simulink model "euler_ZXY_model"  (R2023b)
settings: Solver=FixedStepAuto  StartTime=0.0  StopTime=fs  FixedStep=ts  MaxStep=1e-4  RelTol=1e-3
undefined symbols (not defined in the file): alpha, alpha_1, alpha_2, alpha_d, e1, e2, e3, eta_0, eta_dot_0, f_max, g, gamma, gamma_d, gamma_e, gamma_u, gamma_x, gamma_x1, gamma_x2, J, k_3, k_beta, k_d_gamma, K_p, k_p_gamma, k_R, m, p_0, p_d_0, p_dot_0, p_dot_zmax, r, ts, y_c, z_c, z_dot_max, z_max
libraries: eeGeneralControl x8, slctrl_constraint x6, simulink x2, rbm3d x1, simulink_extras x1
(part 2 of 2)

== system euler_ZXY_model/dynamics/回転方向の運動方程式/Subsystem ==
  M : Inport
  Psi : Inport  Port=2
  tau^b : Inport  Port=3
  C : Inport  Port=4
  eta_dot : Inport  Port=5
  Constant : Constant  Value=e1
  Matrix Multiply : Product  Inputs=3  Multiplication=Matrix(*)
  Matrix Multiply1 : Product  Inputs=3  Multiplication=Matrix(*)
  Matrix Multiply2 : Product  Multiplication=Matrix(*)
  Matrix Multiply3 : Product  Multiplication=Matrix(*)
  Matrix Multiply4 : Product  Multiplication=Matrix(*)
  Product : Product  Inputs=/  Multiplication=Matrix(*)
  Product1 : Product  Inputs=/  Multiplication=Matrix(*)
  Sum : Sum  Inputs=|+-
  Transpose : Math  Operator=transpose
  Transpose1 : Math  Operator=transpose
  lambda_3 : Outport
  wires:
  Constant/1 -> Matrix Multiply/3, Transpose/1
  Transpose/1 -> Matrix Multiply/1, Matrix Multiply1/2
  M/1 -> Product/1
  Product/1 -> Matrix Multiply1/3, Matrix Multiply/2
  Matrix Multiply/1 -> Product1/1
  Product1/1 -> Matrix Multiply1/1
  Matrix Multiply1/1 -> Matrix Multiply2/1
  Matrix Multiply2/1 -> lambda_3/1
  Psi/1 -> Transpose1/1
  Transpose1/1 -> Matrix Multiply3/1
  tau^b/1 -> Matrix Multiply3/2
  Matrix Multiply3/1 -> Sum/1
  C/1 -> Matrix Multiply4/1
  eta_dot/1 -> Matrix Multiply4/2
  Matrix Multiply4/1 -> Sum/2
  Sum/1 -> Matrix Multiply2/2

== system euler_ZXY_model/dynamics/回転方向の運動方程式/eta to R_SO(2) ==
  eta : Inport
  Cos1 : Trigonometry  Operator=cos
  Cos2 : Trigonometry  Operator=cos
  Gain : Gain  Gain=-1
  Matrix Concatenate : Concatenate  Mode=Multidimensional array  ConcatenateDimension=2
  Mux1 : Mux  Inputs=2
  Mux2 : Mux  Inputs=2
  Selector : Selector  InputPortWidth=3  IndexOptions=Index vector (dialog)  Indices=[2]  OutputSizes=1
  Sin1 : Trigonometry
  Sin2 : Trigonometry
  attitude_state : Outport
  wires:
  eta/1 -> Selector/1
  Cos2/1 -> Mux2/2
  Matrix Concatenate/1 -> attitude_state/1
  Mux2/1 -> Matrix Concatenate/2
  Mux1/1 -> Matrix Concatenate/1
  Gain/1 -> Sin2/1
  Cos1/1 -> Mux1/1
  Sin2/1 -> Mux2/1
  Sin1/1 -> Mux1/2
  Selector/1 -> Cos2/1, Gain/1, Cos1/1, Sin1/1  "beta"

== system euler_ZXY_model/Attitude Controller/beta_controller/r_beta/R_tilde ==
  R_d : Inport
  R : Inport  Port=2
  Matrix Multiply : Product  Multiplication=Matrix(*)
  Transpose : Math  Operator=transpose
  R_tilde : Outport
  wires:
  R_d/1 -> Transpose/1
  Transpose/1 -> Matrix Multiply/1
  R/1 -> Matrix Multiply/2
  Matrix Multiply/1 -> R_tilde/1

== system euler_ZXY_model/Attitude Controller/beta_controller/r_beta/r_beta_d ==
  R_d : Inport
  R_d_dot : Inport  Port=2
  Matrix Multiply : Product  Multiplication=Matrix(*)
  Selector : Selector  NumberOfDimensions=2  InputPortWidth=3  IndexOptions=Index vector (dialog),Index vector (dialog)  Indices=[2],1  OutputSizes=1,1
  Transpose : Math  Operator=transpose
  "r_{beta_d}" : Outport
  wires:
  R_d/1 -> Transpose/1
  Transpose/1 -> Matrix Multiply/1
  R_d_dot/1 -> Matrix Multiply/2
  Matrix Multiply/1 -> Selector/1
  Selector/1 -> "r_{beta_d}"/1

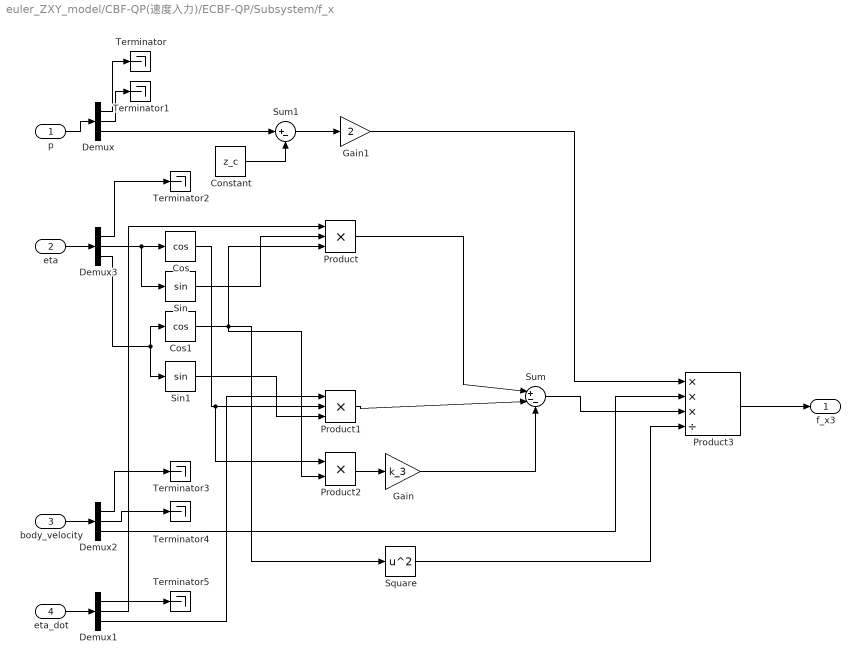
== system euler_ZXY_model/CBF-QP(速度入力)/ECBF-QP/Subsystem/f_x ==
  p : Inport
  eta : Inport  Port=2
  body_velocity : Inport  Port=3
  eta_dot : Inport  Port=4
  Constant : Constant  Value=z_c
  Cos : Trigonometry  Operator=cos
  Cos1 : Trigonometry  Operator=cos
  Demux{,1..3} (4 alike) : Demux  Outputs=3
  Gain : Gain  Gain=k_3
  Gain1 : Gain  Gain=2
  Product : Product  Inputs=3
  Product1 : Product  Inputs=3
  Product2 : Product
  Product3 : Product  Inputs=***/
  Sin : Trigonometry
  Sin1 : Trigonometry
  Square : Math  Operator=square
  Sum : Sum  Inputs=|+--
  Sum1 : Sum  Inputs=|+-
  Terminator{,1..5} (6 alike) : Terminator
  f_x3 : Outport
  wires:
  p/1 -> Demux/1
  Demux/1 -> Terminator/1
  Demux/2 -> Terminator1/1
  eta_dot/1 -> Demux1/1
  body_velocity/1 -> Demux2/1
  eta/1 -> Demux3/1
  Demux3/2 -> Sin/1, Cos/1
  Demux3/3 -> Sin1/1, Cos1/1
  Sin/1 -> Product/2
  Cos1/1 -> Square/1, Product/3, Product2/2
  Demux3/1 -> Terminator2/1
  Demux1/2 -> Product/1
  Demux1/3 -> Product1/1
  Sin1/1 -> Product1/3
  Cos/1 -> Product2/1, Product1/2
  Product2/1 -> Gain/1
  Product1/1 -> Sum/2
  Gain/1 -> Sum/3
  Product/1 -> Sum/1
  Demux/3 -> Sum1/1
  Constant/1 -> Sum1/2
  Sum1/1 -> Gain1/1
  Gain1/1 -> Product3/1
  Demux2/3 -> Product3/2
  Sum/1 -> Product3/3
  Square/1 -> Product3/4
  Product3/1 -> f_x3/1
  Demux2/1 -> Terminator3/1
  Demux2/2 -> Terminator4/1
  Demux1/1 -> Terminator5/1

== system euler_ZXY_model/CBF-QP(速度入力)/ECBF-QP/Subsystem/f_x1 ==
  p_dot : Inport
  Demux : Demux  Outputs=3
  Gain : Gain  Gain=-2
  Square : Math  Operator=square
  Square1 : Math  Operator=square
  Sum : Sum  Inputs=|++
  Terminator : Terminator
  f_x1 : Outport
  wires:
  p_dot/1 -> Demux/1
  Demux/1 -> Terminator/1
  Demux/2 -> Square/1
  Demux/3 -> Square1/1
  Square/1 -> Sum/1
  Square1/1 -> Sum/2
  Sum/1 -> Gain/1
  Gain/1 -> f_x1/1

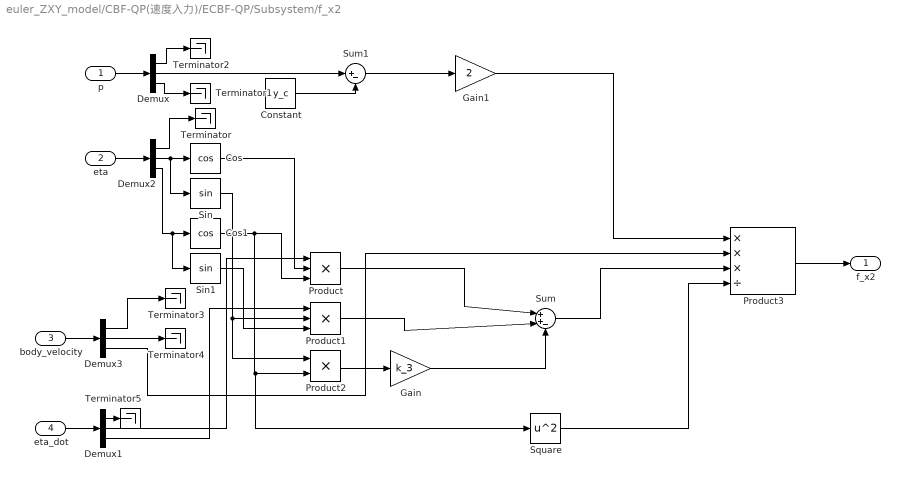
== system euler_ZXY_model/CBF-QP(速度入力)/ECBF-QP/Subsystem/f_x2 ==
  p : Inport
  eta : Inport  Port=2
  body_velocity : Inport  Port=3
  eta_dot : Inport  Port=4
  Constant : Constant  Value=y_c
  Cos : Trigonometry  Operator=cos
  Cos1 : Trigonometry  Operator=cos
  Demux{,1..3} (4 alike) : Demux  Outputs=3
  Gain : Gain  Gain=k_3
  Gain1 : Gain  Gain=2
  Product : Product  Inputs=3
  Product1 : Product  Inputs=3
  Product2 : Product
  Product3 : Product  Inputs=***/
  Sin : Trigonometry
  Sin1 : Trigonometry
  Square : Math  Operator=square
  Sum : Sum  Inputs=|++-
  Sum1 : Sum  Inputs=|+-
  Terminator{,1..5} (6 alike) : Terminator
  f_x2 : Outport
  wires:
  p/1 -> Demux/1
  eta_dot/1 -> Demux1/1
  eta/1 -> Demux2/1
  body_velocity/1 -> Demux3/1
  Demux2/2 -> Sin/1, Cos/1
  Demux2/3 -> Sin1/1, Cos1/1
  Demux2/1 -> Terminator/1
  Cos1/1 -> Square/1, Product2/2, Product/3
  Cos/1 -> Product/2
  Sin1/1 -> Product1/3
  Sin/1 -> Product2/1, Product1/2
  Product2/1 -> Gain/1
  Gain/1 -> Sum/3
  Product1/1 -> Sum/2
  Product/1 -> Sum/1
  Demux/3 -> Terminator1/1
  Demux/1 -> Terminator2/1
  Demux/2 -> Sum1/1
  Constant/1 -> Sum1/2
  Sum1/1 -> Gain1/1
  Gain1/1 -> Product3/1
  Demux1/2 -> Product/1
  Demux1/3 -> Product1/1
  Demux3/3 -> Product3/2
  Sum/1 -> Product3/3
  Square/1 -> Product3/4
  Product3/1 -> f_x2/1
  Demux3/1 -> Terminator3/1
  Demux3/2 -> Terminator4/1
  Demux1/1 -> Terminator5/1

== system euler_ZXY_model/CBF-QP(速度入力)/ECBF-QP/c/Subsystem ==
  p : Inport
  p_dot : Inport  Port=2
  Constant : Constant  Value=y_c
  Constant1 : Constant  Value=z_c
  Demux : Demux  Outputs=3
  Demux1 : Demux  Outputs=3
  Gain : Gain  Gain=2
  Product : Product
  Product1 : Product
  Sum : Sum  Inputs=|+-
  Sum1 : Sum  Inputs=|+-
  Sum2 : Sum  Inputs=|++
  Terminator : Terminator
  Terminator1 : Terminator
  h_dot : Outport
  wires:
  p/1 -> Demux/1
  p_dot/1 -> Demux1/1
  Demux/1 -> Terminator/1
  Demux1/1 -> Terminator1/1
  Demux/2 -> Sum/1
  Constant/1 -> Sum/2
  Sum/1 -> Product/1
  Demux1/2 -> Product/2
  Gain/1 -> h_dot/1
  Product/1 -> Sum2/1
  Sum2/1 -> Gain/1
  Demux/3 -> Sum1/1
  Sum1/1 -> Product1/1
  Constant1/1 -> Sum1/2
  Demux1/3 -> Product1/2
  Product1/1 -> Sum2/2

== system euler_ZXY_model/CBF-QP(速度入力)/ECBF-QP/c/h ==
  p : Inport
  Constant : Constant  Value=y_c
  Constant1 : Constant  Value=r
  Constant2 : Constant  Value=z_c
  Demux : Demux  Outputs=3
  Square : Math  Operator=square
  Square1 : Math  Operator=square
  Sum : Sum  Inputs=|+-
  Sum1 : Sum  Inputs=|+-
  Sum2 : Sum  Inputs=|++-
  Terminator : Terminator
  h : Outport
  wires:
  p/1 -> Demux/1
  Demux/2 -> Sum/1
  Demux/3 -> Sum1/1
  Constant1/1 -> Sum2/3
  Sum2/1 -> h/1
  Sum/1 -> Square/1
  Sum1/1 -> Square1/1
  Square/1 -> Sum2/1
  Square1/1 -> Sum2/2
  Constant/1 -> Sum/2
  Constant2/1 -> Sum1/2
  Demux/1 -> Terminator/1

== system euler_ZXY_model/CBF-QP(速度入力)/ECBF-QP_rengo_ver./c/h ==
  p : Inport
  Constant : Constant  Value=y_c
  Constant1 : Constant  Value=r
  Constant2 : Constant  Value=z_c
  Demux : Demux  Outputs=3
  Square : Math  Operator=square
  Square1 : Math  Operator=square
  Sum : Sum  Inputs=|+-
  Sum1 : Sum  Inputs=|+-
  Sum2 : Sum  Inputs=|++-
  Terminator : Terminator
  h : Outport
  wires:
  p/1 -> Demux/1
  Demux/2 -> Sum/1
  Demux/3 -> Sum1/1
  Constant1/1 -> Sum2/3
  Sum2/1 -> h/1
  Sum/1 -> Square/1
  Sum1/1 -> Square1/1
  Square/1 -> Sum2/1
  Square1/1 -> Sum2/2
  Constant/1 -> Sum/2
  Constant2/1 -> Sum1/2
  Demux/1 -> Terminator/1

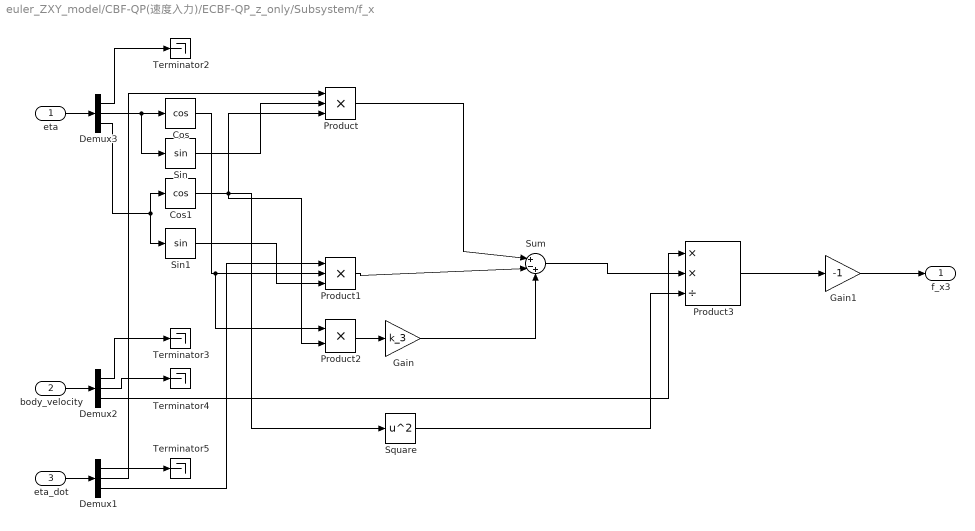
== system euler_ZXY_model/CBF-QP(速度入力)/ECBF-QP_z_only/Subsystem/f_x ==
  eta : Inport
  body_velocity : Inport  Port=2
  eta_dot : Inport  Port=3
  Cos : Trigonometry  Operator=cos
  Cos1 : Trigonometry  Operator=cos
  Demux1 : Demux  Outputs=3
  Demux2 : Demux  Outputs=3
  Demux3 : Demux  Outputs=3
  Gain : Gain  Gain=k_3
  Gain1 : Gain  Gain=-1
  Product : Product  Inputs=3
  Product1 : Product  Inputs=3
  Product2 : Product
  Product3 : Product  Inputs=**/
  Sin : Trigonometry
  Sin1 : Trigonometry
  Square : Math  Operator=square
  Sum : Sum  Inputs=|+-+
  Terminator{2..5} (4 alike) : Terminator
  f_x3 : Outport
  wires:
  eta_dot/1 -> Demux1/1
  body_velocity/1 -> Demux2/1
  eta/1 -> Demux3/1
  Demux3/2 -> Sin/1, Cos/1
  Demux3/3 -> Sin1/1, Cos1/1
  Sin/1 -> Product/2
  Cos1/1 -> Square/1, Product/3, Product2/2
  Demux3/1 -> Terminator2/1
  Demux1/2 -> Product/1
  Demux1/3 -> Product1/1
  Sin1/1 -> Product1/3
  Cos/1 -> Product2/1, Product1/2
  Product2/1 -> Gain/1
  Product1/1 -> Sum/2
  Gain/1 -> Sum/3
  Product/1 -> Sum/1
  Demux2/3 -> Product3/1
  Sum/1 -> Product3/2
  Square/1 -> Product3/3
  Demux2/1 -> Terminator3/1
  Demux2/2 -> Terminator4/1
  Demux1/1 -> Terminator5/1
  Product3/1 -> Gain1/1
  Gain1/1 -> f_x3/1

== system euler_ZXY_model/CBF-QP(速度入力)/ECBF-QP_z_only/c/Subsystem ==
  p_dot : Inport
  Demux1 : Demux  Outputs=3
  Gain : Gain  Gain=-1
  Terminator1 : Terminator
  Terminator2 : Terminator
  h_dot : Outport
  wires:
  p_dot/1 -> Demux1/1
  Demux1/1 -> Terminator1/1
  Gain/1 -> h_dot/1
  Demux1/2 -> Terminator2/1
  Demux1/3 -> Gain/1

== system euler_ZXY_model/CBF-QP(速度入力)/ECBF-QP_z_only/c/h ==
  p : Inport
  Constant2 : Constant  Value=z_c
  Demux : Demux  Outputs=3
  Gain : Gain  Gain=-1
  Sum1 : Sum  Inputs=|+-
  Terminator : Terminator
  Terminator1 : Terminator
  h : Outport
  wires:
  p/1 -> Demux/1
  Demux/2 -> Terminator1/1
  Demux/3 -> Sum1/1
  Gain/1 -> h/1
  Sum1/1 -> Gain/1
  Constant2/1 -> Sum1/2
  Demux/1 -> Terminator/1

== system euler_ZXY_model/dynamics/並進方向の運動方程式/B/Subsystem ==
  R : Inport
  Constant1 : Constant  Value=0
  Selector : Selector  NumberOfDimensions=2  InputPortWidth=3  IndexOptions=Index vector (dialog),Index vector (dialog)  Indices=[2],[2]  OutputSizes=1,1
  Selector1 : Selector  NumberOfDimensions=2  InputPortWidth=3  IndexOptions=Index vector (dialog),Index vector (dialog)  Indices=[3],[2]  OutputSizes=1,1
  Transpose : Math  Operator=transpose
  Vector Concatenate : Concatenate  NumInputs=3
  A : Outport
  wires:
  R/1 -> Selector1/1, Selector/1
  Selector/1 -> Vector Concatenate/2
  Selector1/1 -> Vector Concatenate/3
  Constant1/1 -> Vector Concatenate/1
  Vector Concatenate/1 -> Transpose/1
  Transpose/1 -> A/1

== system euler_ZXY_model/dynamics/並進方向の運動方程式/Rotation matrix_ZXY/R1 ==
  In1 : Inport
  Cos : Trigonometry  Operator=cos
  Cos1 : Trigonometry  Operator=cos
  Cos2 : Trigonometry  Operator=cos
  Demux : Demux  Outputs=3
  Gain : Gain  Gain=-1
  Matrix Concatenate : Concatenate  NumInputs=3
  Product : Product
  Product1 : Product  Inputs=3
  Product2 : Product
  Product3 : Product  Inputs=3
  Product4 : Product
  Sin : Trigonometry
  Sin1 : Trigonometry
  Sin2 : Trigonometry
  Sum : Sum  Inputs=|+-
  Sum1 : Sum  Inputs=|++
  Out1 : Outport  VectorParamsAs1DForOutWhenUnconnected=off
  wires:
  Matrix Concatenate/1 -> Out1/1
  In1/1 -> Demux/1
  Demux/3 -> Sin/1, Cos/1
  Demux/2 -> Sin1/1, Cos1/1
  Demux/1 -> Cos2/1, Sin2/1
  Cos2/1 -> Product3/1, Product/1
  Cos/1 -> Product2/2, Product/2
  Product/1 -> Sum/1
  Sin2/1 -> Product2/1, Product1/1
  Sin1/1 -> Product3/2, Product1/2
  Sin/1 -> Product3/3, Product1/3, Product4/2
  Product1/1 -> Sum/2
  Product2/1 -> Sum1/1
  Product3/1 -> Sum1/2
  Cos1/1 -> Product4/1
  Product4/1 -> Gain/1
  Sum1/1 -> Matrix Concatenate/2
  Gain/1 -> Matrix Concatenate/3
  Sum/1 -> Matrix Concatenate/1

== system euler_ZXY_model/dynamics/並進方向の運動方程式/Rotation matrix_ZXY/R2 ==
  In1 : Inport
  Cos1 : Trigonometry  Operator=cos
  Cos2 : Trigonometry  Operator=cos
  Demux : Demux  Outputs=3
  Gain : Gain  Gain=-1
  Matrix Concatenate : Concatenate  NumInputs=3
  Product : Product
  Product1 : Product
  Sin1 : Trigonometry
  Sin2 : Trigonometry
  Terminator : Terminator
  Out1 : Outport  VectorParamsAs1DForOutWhenUnconnected=off
  wires:
  In1/1 -> Demux/1
  Demux/2 -> Cos1/1, Sin1/1
  Matrix Concatenate/1 -> Out1/1
  Demux/1 -> Cos2/1, Sin2/1
  Sin2/1 -> Product/1
  Cos1/1 -> Product/2, Product1/2
  Product/1 -> Gain/1
  Cos2/1 -> Product1/1
  Gain/1 -> Matrix Concatenate/1
  Product1/1 -> Matrix Concatenate/2
  Sin1/1 -> Matrix Concatenate/3
  Demux/3 -> Terminator/1

== system euler_ZXY_model/dynamics/並進方向の運動方程式/Rotation matrix_ZXY/R3 ==
  In1 : Inport
  Cos1 : Trigonometry  Operator=cos
  Cos2 : Trigonometry  Operator=cos
  Cos3 : Trigonometry  Operator=cos
  Demux : Demux  Outputs=3
  Matrix Concatenate : Concatenate  NumInputs=3
  Product : Product
  Product1 : Product  Inputs=3
  Product2 : Product
  Product3 : Product  Inputs=3
  Product4 : Product
  Sin1 : Trigonometry
  Sin2 : Trigonometry
  Sin3 : Trigonometry
  Sum : Sum  Inputs=|++
  Sum1 : Sum  Inputs=|+-
  Out1 : Outport  VectorParamsAs1DForOutWhenUnconnected=off
  wires:
  Matrix Concatenate/1 -> Out1/1
  Demux/2 -> Sin1/1, Cos1/1
  Demux/3 -> Sin2/1, Cos2/1
  In1/1 -> Demux/1
  Cos2/1 -> Product4/2, Product3/3, Product1/3
  Demux/1 -> Cos3/1, Sin3/1
  Cos3/1 -> Product3/1, Product/1
  Sin2/1 -> Product2/2, Product/2
  Product/1 -> Sum/1
  Sin3/1 -> Product2/1, Product1/1
  Sin1/1 -> Product3/2, Product1/2
  Product1/1 -> Sum/2
  Product2/1 -> Sum1/1
  Product3/1 -> Sum1/2
  Cos1/1 -> Product4/1
  Sum/1 -> Matrix Concatenate/1
  Sum1/1 -> Matrix Concatenate/2
  Product4/1 -> Matrix Concatenate/3

== system euler_ZXY_model/dynamics/回転方向の運動方程式/C(η,η_dot)/skew ==
  Ψ(η) : Inport
  eta_dot : Inport  Port=2
  3D wedge : rbm3d/3D wedge
  Product : Product  Multiplication=Matrix(*)
  skew(Ω) : Outport  VectorParamsAs1DForOutWhenUnconnected=off
  wires:
  eta_dot/1 -> Product/2
  Product/1 -> 3D wedge/1
  3D wedge/1 -> skew(Ω)/1
  Ψ(η)/1 -> Product/1

== system euler_ZXY_model/dynamics/回転方向の運動方程式/Euler_matrix_ZXY/Psi_*1 ==
  eta : Inport
  Cos : Trigonometry  Operator=cos
  Cos1 : Trigonometry  Operator=cos
  Demux : Demux  Outputs=3
  Gain : Gain  Gain=-1
  Product : Product
  Product1 : Product
  Sin : Trigonometry
  Sin1 : Trigonometry
  Terminator : Terminator
  Vector Concatenate : Concatenate  NumInputs=3
  Out1 : Outport
  wires:
  eta/1 -> Demux/1
  Demux/1 -> Terminator/1
  Demux/2 -> Cos/1, Sin1/1
  Demux/3 -> Cos1/1, Sin/1
  Cos/1 -> Product1/1, Product/1
  Sin/1 -> Product/2
  Product/1 -> Vector Concatenate/1
  Sin1/1 -> Gain/1
  Gain/1 -> Vector Concatenate/2
  Vector Concatenate/1 -> Out1/1
  Cos1/1 -> Product1/2
  Product1/1 -> Vector Concatenate/3

== system euler_ZXY_model/dynamics/回転方向の運動方程式/Euler_matrix_ZXY/Psi_*2 ==
  eta : Inport
  Constant : Constant  Value=0
  Cos : Trigonometry  Operator=cos
  Demux : Demux  Outputs=3
  Gain : Gain  Gain=-1
  Sin : Trigonometry
  Terminator : Terminator
  Terminator1 : Terminator
  Vector Concatenate : Concatenate  NumInputs=3
  Out1 : Outport
  wires:
  eta/1 -> Demux/1
  Demux/1 -> Terminator/1
  Demux/2 -> Terminator1/1
  Demux/3 -> Sin/1, Cos/1
  Sin/1 -> Gain/1
  Cos/1 -> Vector Concatenate/1
  Constant/1 -> Vector Concatenate/2
  Gain/1 -> Vector Concatenate/3
  Vector Concatenate/1 -> Out1/1

== system euler_ZXY_model/dynamics/回転方向の運動方程式/Rotation matrix_ZXY/R1 ==
  In1 : Inport
  Cos : Trigonometry  Operator=cos
  Cos1 : Trigonometry  Operator=cos
  Cos2 : Trigonometry  Operator=cos
  Demux : Demux  Outputs=3
  Gain : Gain  Gain=-1
  Matrix Concatenate : Concatenate  NumInputs=3
  Product : Product
  Product1 : Product  Inputs=3
  Product2 : Product
  Product3 : Product  Inputs=3
  Product4 : Product
  Sin : Trigonometry
  Sin1 : Trigonometry
  Sin2 : Trigonometry
  Sum : Sum  Inputs=|+-
  Sum1 : Sum  Inputs=|++
  Out1 : Outport  VectorParamsAs1DForOutWhenUnconnected=off
  wires:
  Matrix Concatenate/1 -> Out1/1
  In1/1 -> Demux/1
  Demux/3 -> Sin/1, Cos/1
  Demux/2 -> Sin1/1, Cos1/1
  Demux/1 -> Cos2/1, Sin2/1
  Cos2/1 -> Product3/1, Product/1
  Cos/1 -> Product2/2, Product/2
  Product/1 -> Sum/1
  Sin2/1 -> Product2/1, Product1/1
  Sin1/1 -> Product3/2, Product1/2
  Sin/1 -> Product3/3, Product1/3, Product4/2
  Product1/1 -> Sum/2
  Product2/1 -> Sum1/1
  Product3/1 -> Sum1/2
  Cos1/1 -> Product4/1
  Product4/1 -> Gain/1
  Sum1/1 -> Matrix Concatenate/2
  Gain/1 -> Matrix Concatenate/3
  Sum/1 -> Matrix Concatenate/1

== system euler_ZXY_model/dynamics/回転方向の運動方程式/Rotation matrix_ZXY/R2 ==
  In1 : Inport
  Cos1 : Trigonometry  Operator=cos
  Cos2 : Trigonometry  Operator=cos
  Demux : Demux  Outputs=3
  Gain : Gain  Gain=-1
  Matrix Concatenate : Concatenate  NumInputs=3
  Product : Product
  Product1 : Product
  Sin1 : Trigonometry
  Sin2 : Trigonometry
  Terminator : Terminator
  Out1 : Outport  VectorParamsAs1DForOutWhenUnconnected=off
  wires:
  In1/1 -> Demux/1
  Demux/2 -> Cos1/1, Sin1/1
  Matrix Concatenate/1 -> Out1/1
  Demux/1 -> Cos2/1, Sin2/1
  Sin2/1 -> Product/1
  Cos1/1 -> Product/2, Product1/2
  Product/1 -> Gain/1
  Cos2/1 -> Product1/1
  Gain/1 -> Matrix Concatenate/1
  Product1/1 -> Matrix Concatenate/2
  Sin1/1 -> Matrix Concatenate/3
  Demux/3 -> Terminator/1

== system euler_ZXY_model/dynamics/回転方向の運動方程式/Rotation matrix_ZXY/R3 ==
  In1 : Inport
  Cos1 : Trigonometry  Operator=cos
  Cos2 : Trigonometry  Operator=cos
  Cos3 : Trigonometry  Operator=cos
  Demux : Demux  Outputs=3
  Matrix Concatenate : Concatenate  NumInputs=3
  Product : Product
  Product1 : Product  Inputs=3
  Product2 : Product
  Product3 : Product  Inputs=3
  Product4 : Product
  Sin1 : Trigonometry
  Sin2 : Trigonometry
  Sin3 : Trigonometry
  Sum : Sum  Inputs=|++
  Sum1 : Sum  Inputs=|+-
  Out1 : Outport  VectorParamsAs1DForOutWhenUnconnected=off
  wires:
  Matrix Concatenate/1 -> Out1/1
  Demux/2 -> Sin1/1, Cos1/1
  Demux/3 -> Sin2/1, Cos2/1
  In1/1 -> Demux/1
  Cos2/1 -> Product4/2, Product3/3, Product1/3
  Demux/1 -> Cos3/1, Sin3/1
  Cos3/1 -> Product3/1, Product/1
  Sin2/1 -> Product2/2, Product/2
  Product/1 -> Sum/1
  Sin3/1 -> Product2/1, Product1/1
  Sin1/1 -> Product3/2, Product1/2
  Product1/1 -> Sum/2
  Product2/1 -> Sum1/1
  Product3/1 -> Sum1/2
  Cos1/1 -> Product4/1
  Sum/1 -> Matrix Concatenate/1
  Sum1/1 -> Matrix Concatenate/2
  Product4/1 -> Matrix Concatenate/3

== matlab function euler_ZXY_model/Velocity Feedback Controller/MATLAB Function6 ==
  data: R input; v input; omega input; F output size=1; u_3 input; du_3 input; k_3 parameter; g parameter; m parameter
function F = fcn(R,v,omega,u_3,du_3,k_3, g, m)

F1 = (1 - (R(1,3)*(R(3,2)*R(2,1) - R(2,2)*R(3,1)))/(R(1,1)*(R(3,2)*R(2,3) - R(2,2)*R(3,3))))*( -k_3*( v(3,1) - u_3) + du_3 );
F2 = ( v(3,1)*omega(2,1)*(R(3,2)*R(2,1)-R(2,2)*R(3,1) ) - g*R(1,1)*R(2,2) + omega(2,1)*R(1,3)*v(1,1) - omega(2,1)*R(1,1)*v(3,1) )/(R(1,1)*(R(3,2)*R(2,3) - R(2,2)*R(3,3)));
F3 = -v(1,1)*omega(2,1);

F = m*(F1 + F2 + F3);

% F = m((1 - (R(1,3)*(R(3,2)*R(2,1) - R(2,2)*R(3,1)))/(R(1,1)*(R(3,2)*R(2,3) - R(2,2)*R(3,3))))*k_3*(u_3 - v(3,1)) + ((-v(2,1)*omega(3,1) + v(3,1)*omega(2,1))*(R(3,2)*R(2,1) - R(2,2)*R(3,1)) - g*R(2,2))/(R(3,2)*R(2,3) - R(2,2)*R(3,3)) + (-v(1,1)*omega(2,1) + v(2,1)*omega(1,1)));
% F2 = ((-v(2,1)*omega(3,1) + v(3,1)*omega(2,1))*(R(3,2)*R(2,1) - R(2,2)*R(3,1)) - g*R(2,2))/(R(3,2)*R(2,3) - R(2,2)*R(3,3));
% F3 = -v(1,1)*omega(2,1) + v(2,1)*omega(1,1);

== matlab function euler_ZXY_model/I-CBF(推力修正型)/MATLAB Function6 ==
  settings: updateMethod=DISCRETE  sampleTime=ts
  data: R input; v input; omega input; g parameter; f output size=3
function f  = fcn(R,v,omega, g)

f1 = 1 - (R(1,3)*( R(3,2)*R(2,1) - R(2,2)*R(3,1) ) )/(R(1,1)*(R(3,2)*R(2,3) - R(2,2)*R(3,3)));
f2 = ( v(3,1)*omega(2,1)*(R(3,2)*R(2,1)-R(2,2)*R(3,1) ) - g*R(1,1)*R(2,2) + omega(2,1)*R(1,3)*v(1,1) - omega(2,1)*R(1,1)*v(3,1) )/(R(1,1)*(R(3,2)*R(2,3) - R(2,2)*R(3,3)) );
f3 = -v(1,1)*omega(2,1);
f = [f1;f2;f3];

== matlab function euler_ZXY_model/I-CBF(推力修正型)/MATLAB Function1 ==
  data: R input; v input; omega input; F output size=1; u_3 input; du_3 input; k_3 parameter; g parameter; m parameter
function F = fcn(R,v,omega,u_3,du_3,k_3, g, m)

F1 = (1 - (R(1,3)*(R(3,2)*R(2,1) - R(2,2)*R(3,1)))/(R(1,1)*(R(3,2)*R(2,3) - R(2,2)*R(3,3))))*( -k_3*( v(3,1) - u_3) + du_3 );
F2 = ( v(3,1)*omega(2,1)*(R(3,2)*R(2,1)-R(2,2)*R(3,1) ) - g*R(1,1)*R(2,2) + omega(2,1)*R(1,3)*v(1,1) - omega(2,1)*R(1,1)*v(3,1) )/(R(1,1)*(R(3,2)*R(2,3) - R(2,2)*R(3,3)));
F3 = -v(1,1)*omega(2,1);

F = m*(F1 + F2 + F3);

% F = m((1 - (R(1,3)*(R(3,2)*R(2,1) - R(2,2)*R(3,1)))/(R(1,1)*(R(3,2)*R(2,3) - R(2,2)*R(3,3))))*k_3*(u_3 - v(3,1)) + ((-v(2,1)*omega(3,1) + v(3,1)*omega(2,1))*(R(3,2)*R(2,1) - R(2,2)*R(3,1)) - g*R(2,2))/(R(3,2)*R(2,3) - R(2,2)*R(3,3)) + (-v(1,1)*omega(2,1) + v(2,1)*omega(1,1)));
% F2 = ((-v(2,1)*omega(3,1) + v(3,1)*omega(2,1))*(R(3,2)*R(2,1) - R(2,2)*R(3,1)) - g*R(2,2))/(R(3,2)*R(2,3) - R(2,2)*R(3,3));
% F3 = -v(1,1)*omega(2,1) + v(2,1)*omega(1,1);

== stateflow chart euler_ZXY_model/reference/y_d_dot ==
  state transition_state
    entry:
    y_d_dot = 0.3*15*pi/180;
    during:
    y_d_dot = 0.3*(15*pi/180)*cos(15*pi*t/180);
  state steady_state
    entry: y_d_dot = 0;
  (default) -> transition_state : []
  transition_state -> steady_state : [t >= 6]
  data: t input; y_d_dot output

== matlab function euler_ZXY_model/CBF(通常ドローンホバリングの推力入力)/MATLAB Function ==
  data: z input; z_dot input; rot input; fx output; gx output; c output; m parameter; alpha_1 parameter; alpha_2 parameter; g parameter; z_c parameter; lambda1 input
function [fx,gx,c]= fcn(z,z_dot, rot, m, alpha_1, alpha_2, g, z_c, lambda1)

%各要素に名前を付ける 

r32 = rot(3,2);
r33 = rot(3,3);


%CBF関数h(3回微分まで使う)
h = z_c - z;
h_dot = - z_dot;

%出力
fx = - g - (lambda1*r32/m);

gx = r33/m;
     
c = alpha_1*h + alpha_2*h_dot;

== matlab function euler_ZXY_model/I-CBF/MATLAB Function ==
  data: phi input; p input; p_dot input; p_ddot input; R input; gamma_u parameter; f_max parameter; m parameter; gamma_x parameter; f output; g output; R_dot input; p_dot_zmax parameter; gamma_e parameter; gamma_x1 parameter; gamma_x2 parameter; z_max parameter; lambda_1 input; lambda_dot_1 input; u input
function [f,g] = fcn(phi, p, p_dot, p_ddot, R, gamma_u, f_max, m, gamma_x, R_dot, p_dot_zmax, gamma_e, gamma_x1, gamma_x2, z_max,lambda_1,lambda_dot_1, u)

%推力制約に関わる部分%
h_u = f_max - u^2;
fu = 2*u*phi - gamma_u*h_u;
gu = 2*u;      

% パラメータ
r_32 = R(3,2);
r_33 = R(3,3);
r_dot_32 = R_dot(3,2);
r_dot_33 = R_dot(3,3);
p_dot_z = p_dot(3);
p_ddot_z = p_ddot(3);
z = p(3);
z_dot = p_dot(3);
z_ddot = p_ddot(3);
h_e = - z_ddot - gamma_x1*z_dot + gamma_x2*(z_max - z);

%速度制約に関わる部分%
% fx = -gamma_e*(- p_ddot_z + gamma_x*(p_dot_zmax - p_dot_z)) -(lambda_dot_1/m)*r_32 - (lambda_1/m)*r_dot_32+ (r_dot_33/m)*u + (r_33/m)*phi + gamma_x*p_ddot_z;
% gx = r_33/m;

% %位置制約に関わる部分%
fx = - gamma_e*h_e -(1/m)*lambda_dot_1*r_32 - (1/m)*lambda_1*r_dot_32 + (1/m)*phi*r_33 + (u/m)*r_dot_33 + gamma_x1*z_ddot + gamma_x2*z_dot;
gx = r_33/m;


f = [fx;fu];
g = [gx;gu];
% fx = fv;
% gx = gv;
